simulink model "MRR_H8"  (R2025a)
settings: Solver=VariableStepAuto  StartTime=0.0  StopTime=20.0  MaxStep=1/25  RelTol=1e-3
InitFcn:
  | K = 1;
  | tau = 1;
  | xi = 0.25;
settings Model: Creator=Szalay  LastModifiedBy=Szalay

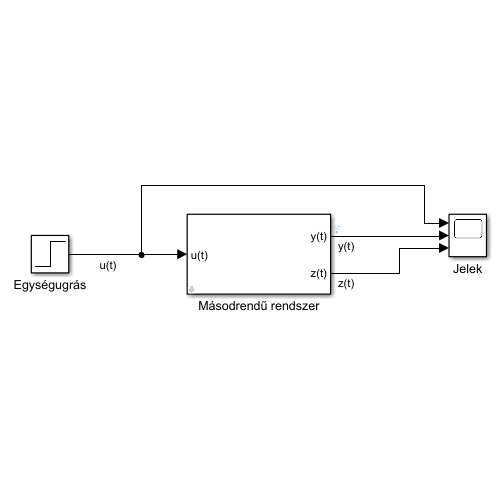
[thumbnail: Simulink's stored preview of the top-level diagram]
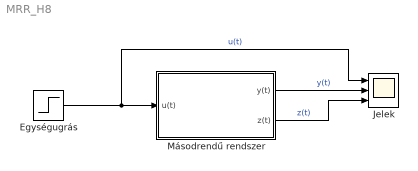
== system MRR_H8 ==
  Egységugrás : Step  SampleTime=0
  Jelek : Scope  NumInputPorts=3
      settings: ActiveDisplayYMinimum=-0.24999997198601773  ActiveDisplayYMaximum=2.2499997478741602
  Másodrendű rendszer : Subsystem  mask(Másodrendű rendszer){K=K, tau=tau, xi=xi, y_0=0, z_0=0}
      mask prompts: K "Állandósult állapoti erősítés"; tau "Időállandó (s)"; xi "Csillapítási tényező"; y_0 "A kimenet kezdeti értéke"; z_0 "A kimenet deriváltjának kezdeti értéke"
      mask help: A lineáris közönséges másodfokú differenciálegyenlet leképezése.
      mask DialogControl ParameterGroupVar Prompt: Rendszerparaméterek
      mask DialogControl Container3 Prompt: Kezdeti értékek
  wires:
  Egységugrás/1 -> Jelek/1, Másodrendű rendszer/1(u(t))  "u(t)"
  Másodrendű rendszer/1(y(t)) -> Jelek/2  "y(t)"
  Másodrendű rendszer/2(z(t)) -> Jelek/3  "z(t)"

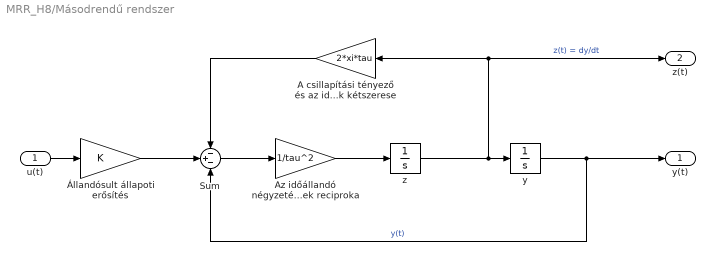
== system MRR_H8/Másodrendű rendszer ==
  u(t) : Inport
  A csillapítási tényező és az időállandó szorzatának kétszerese : Gain  Gain=2*xi*tau
  Az időállandó négyzetének reciproka : Gain  Gain=1/tau^2
  Sum : Sum  Inputs=-+-
  y : Integrator  InitialCondition=y_0
  z : Integrator  InitialCondition=z_0
  Állandósult állapoti erősítés : Gain  Gain=K
  y(t) : Outport
  z(t) : Outport  Port=2
  wires:
  A csillapítási tényező és az időállandó szorzatának kétszerese/1 -> Sum/1
  z/1 -> A csillapítási tényező és az időállandó szorzatának kétszerese/1, z(t)/1, y/1  "z(t) = dy/dt"
  Az időállandó négyzetének reciproka/1 -> z/1
  Sum/1 -> Az időállandó négyzetének reciproka/1
  y/1 -> y(t)/1, Sum/3  "y(t)"
  Állandósult állapoti erősítés/1 -> Sum/2
  u(t)/1 -> Állandósult állapoti erősítés/1
